simulink model "simulation"  (R2018b)
settings: Solver=FixedStepDiscrete  StartTime=0.0  StopTime=simtime  FixedStep=stepsize  RelTol=1e-3
undefined symbols (not defined in the file): activate_stop, activate_stop_vmax, ay_stop, Bat_param, deltav_ist, DiscIntNeverNeededParam, EG_wunsch, magnitude, mu_road_LF, mu_road_LR, mu_road_RF, mu_road_RR, par_ASR, par_MDT, par_TIR, par_VEH, select_delta_h, select_M_wheel, stepsize, t, temp_betriebsstrategie, temperature_LTrange, track_left, track_right
libraries: Library_ASK x36, simulink x18, dspstat3 x2, Library_Betriebsstrategie x2, vehicle_model x2, pacejka_trans x1
(part 4 of 6)

== system simulation/Vehicle/Antriebsstrang und Radmomentenverteilung/Drehzahlrückführung az VA/Verzögerungsglied ==
  M : Inport
  IC : InitialCondition  Value=0
  PT1_VA : DiscreteTransferFcn  Numerator=par_VEH.dt.other.PT_Num  Denominator=par_VEH.dt.other.PT_Denom
  Zero-Order Hold : ZeroOrderHold  SampleTime=stepsize
  M_d : Outport
  wires:
  IC/1 -> M_d/1
  PT1_VA/1 -> IC/1
  M/1 -> Zero-Order Hold/1
  Zero-Order Hold/1 -> PT1_VA/1

== system simulation/Vehicle/Betriebsstrategie/Momentenverteilung_und_Schaltstrategie1/ASR ==
  Input : Inport
  Limits_In : Inport  Port=2
  mu_road : Inport  Port=3
  Bus Creator : BusCreator  Inputs=10
  Bus Selector : BusSelector  OutputSignals=Fx_RF_ub,Fx_LF_ub,Fx_RR_ub,Fx_LR_ub
  Bus Selector1 : BusSelector  OutputSignals=kappa.kappa_RF,kappa.kappa_LF,kappa.kappa_RR,kappa.kappa_LR
  Bus Selector2 : BusSelector  OutputSignals=x.vx
  Bus Selector3 : BusSelector  OutputSignals=Fz.Fz_RF,Fz.Fz_LF,Fz.Fz_RR,Fz.Fz_LR
  Bus Selector4 : BusSelector  OutputSignals=mu_road_RF,mu_road_LF,mu_road_RR,mu_road_LR
  Bus Selector6 : BusSelector  OutputSignals=Fx_RF_lb,Fx_LF_lb,Fx_RR_lb,Fx_LR_lb,a_f,a_r
  Constant : Constant  Value=0
  Constant1 : Constant  Value=0
  Constant2 : Constant
  Demux : Demux
  Gain : Gain  Gain=500
  Gain1 : Gain  Gain=1/2000
  Gain2 : Gain
  Math Function : Math  Operator=square  SaturateOnIntegerOverflow=on
  Mux : Mux
  Mux1 : Mux
  Mux2 : Mux
  Product : Product
  Saturation1 : Saturate  UpperLimit=1000  LowerLimit=0
  Scope2 : Scope
  Subtract : Sum  Inputs=-+
  Subtract1 : Sum  Inputs=-+
  Switch : Switch  Criteria=u2 > Threshold
  Switch1 : Switch  Criteria=u2 > Threshold
  opt Schlupf : Subsystem
  Limits_Out : Outport
  wires:
  Gain1/1 -> Subtract1/1
  Saturation1/1 -> Gain1/1
  Product/1 -> Demux/1
  Constant1/1 -> Switch1/3
  Switch1/1 -> Saturation1/1
  Bus Selector2/1 -> Switch1/2  "<vx>"
  Math Function/1 -> Switch1/1
  Gain/1 -> Math Function/1
  Switch/1 -> Gain/1
  Constant/1 -> Switch/3
  Bus Selector1/4 -> Mux/4  "<kappa_LR>"
  Bus Selector1/3 -> Mux/3  "<kappa_RR>"
  Bus Selector1/2 -> Mux/2  "<kappa_LF>"
  Bus Selector1/1 -> Mux/1  "<kappa_RF>"
  Limits_In/1 -> Bus Selector/1, Bus Selector6/1
  mu_road/1 -> Bus Selector4/1
  Bus Selector4/1 -> opt Schlupf/1(mu_RF)  "<mu_road_RF>"
  Bus Selector3/1 -> opt Schlupf/5(Fz_RF)  "<Fz_RF>"
  Bus Selector4/2 -> opt Schlupf/2(mu_LF)  "<mu_road_LF>"
  Bus Selector4/3 -> opt Schlupf/3(mu_RR)  "<mu_road_RR>"
  Bus Selector3/2 -> opt Schlupf/6(Fz_LF)  "<Fz_LF>"
  Bus Selector3/4 -> opt Schlupf/8(Fz_LR)  "<Fz_LR>"
  opt Schlupf/1(kappa_soll_RF) -> Mux2/1
  opt Schlupf/2(kappa_soll_LF) -> Mux2/2
  opt Schlupf/3(kappa_soll_RR) -> Mux2/3
  opt Schlupf/4(kappa_soll_LR) -> Mux2/4
  Mux2/1 -> Gain2/1
  Subtract/1 -> Switch/2, Switch/1
  Bus Selector4/4 -> opt Schlupf/4(mu_LR)  "<mu_road_LR>"
  Bus Selector3/3 -> opt Schlupf/7(Fz_RR)  "<Fz_RR>"
  Input/1 -> Bus Selector3/1, Bus Selector2/1, Bus Selector1/1
  Mux/1 -> Subtract/2
  Mux1/1 -> Product/2
  Bus Selector/1 -> Mux1/1  "<Fx_RF_ub>"
  Bus Selector/2 -> Mux1/2  "<Fx_LF_ub>"
  Bus Selector/3 -> Mux1/3  "<Fx_RR_ub>"
  Bus Selector/4 -> Mux1/4  "<Fx_LR_ub>"
  Demux/1 -> Bus Creator/1  "Fx_RF_ub"
  Demux/2 -> Bus Creator/2  "Fx_LF_ub"
  Demux/3 -> Bus Creator/3  "Fx_RR_ub"
  Demux/4 -> Scope2/1, Bus Creator/4  "Fx_LR_ub"
  Bus Selector6/5 -> Bus Creator/9  "<a_f>"
  Bus Selector6/6 -> Bus Creator/10  "<a_r>"
  Bus Creator/1 -> Limits_Out/1
  Subtract1/1 -> Product/1
  Constant2/1 -> Subtract1/2
  Gain2/1 -> Subtract/1
  Bus Selector6/1 -> Bus Creator/5  "<Fx_RF_lb>"
  Bus Selector6/2 -> Bus Creator/6  "<Fx_LF_lb>"
  Bus Selector6/3 -> Bus Creator/7  "<Fx_RR_lb>"
  Bus Selector6/4 -> Bus Creator/8  "<Fx_LR_lb>"

== system simulation/Vehicle/Betriebsstrategie/Momentenverteilung_und_Schaltstrategie1/Feedback Controller ==
  Input : Inport
  Gierrate ref : Inport  Port=2
  Bus Selector2 : BusSelector  OutputSignals=psi.psip
  Feedback control gain : Gain  Gain=par_VEH.tv_control
  Sum : Sum  Inputs=|+-
  M_z_FB : Outport
  wires:
  Bus Selector2/1 -> Sum/2  "<psip>"
  Input/1 -> Bus Selector2/1
  Feedback control gain/1 -> M_z_FB/1
  Sum/1 -> Feedback control gain/1  "error"
  Gierrate ref/1 -> Sum/1

== system simulation/Vehicle/Betriebsstrategie/Momentenverteilung_und_Schaltstrategie1/Feedforward Controller ==
  Input : Inport
  Gierrate ref : Inport  Port=2
  Add : Sum  Inputs=++++
  Add1 : Sum  Inputs=--
  Add2 : Sum
  Add4 : Sum  Inputs=+-
  Add5 : Sum
  Add6 : Sum
  Bus Selector2 : BusSelector  OutputSignals=x.vx,beta.beta,delta_kinematic.delta_RF,delta_kinematic.delta_LF,delta_kinematic.delta_RR,delta_kinematic.delta_LR
  Compare To Zero : simulink/Logic and Bit Operations/Compare To Zero  relop===  OutDataTypeStr=boolean
  Constant1 : Constant  Value=par_VEH.Iz
  Constant10 : Constant  Value=par_VEH.cornering_stiffness_R
  Constant5 : Constant  Value=0
  Constant6 : Constant  Value=0
  Constant7 : Constant  Value=par_VEH.lF
  Constant8 : Constant  Value=par_VEH.lR
  Constant9 : Constant  Value=par_VEH.cornering_stiffness_F
  Discrete Derivative : simulink/Discrete/Discrete Derivative  gainval=1.0  ICPrevScaledInput=0.0  OutMin=[]  OutMax=[]  OutDataType=fixdt(1, 16)  OutScaling=2^-10  DoSatur=off
  Divide{1,6,9..14} (8 alike) : Product  Inputs=**
  Divide7 : Product  Inputs=*/
  Divide8 : Product  Inputs=***
  Gain1 : Gain  Gain=-1
  Gain2 : Gain  Gain=0.5
  Gain3 : Gain  Gain=0.5
  Math Function : Math  Operator=square  SaturateOnIntegerOverflow=on
  Math Function1 : Math  Operator=square  SaturateOnIntegerOverflow=on
  Saturation : Saturate  UpperLimit=1000
  Switch : Switch  Criteria=u2 > Threshold
  M_z_FF : Outport
  wires:
  Input/1 -> Bus Selector2/1
  Gierrate ref/1 -> Divide7/1, Discrete Derivative/1
  Discrete Derivative/1 -> Divide1/2
  Constant1/1 -> Divide1/1
  Divide1/1 -> Divide6/1
  Bus Selector2/1 -> Divide7/2, Compare To Zero/1  "<vx>"
  Constant5/1 -> Divide6/2
  Divide6/1 -> Saturation/1
  Saturation/1 -> Add/1
  Compare To Zero/1 -> Switch/2
  Constant6/1 -> Switch/1
  Divide7/1 -> Switch/3
  Constant9/1 -> Divide12/2, Divide9/2, Divide8/3
  Constant8/1 -> Math Function1/1, Divide10/1
  Constant10/1 -> Divide13/1, Divide10/2
  Bus Selector2/2 -> Divide11/2  "<beta>"
  Divide10/1 -> Add4/2
  Divide9/1 -> Add4/1
  Add4/1 -> Divide11/1
  Constant7/1 -> Math Function/1, Divide9/1, Divide8/2
  Math Function/1 -> Divide12/1
  Math Function1/1 -> Divide13/2
  Divide13/1 -> Add5/2
  Divide12/1 -> Add5/1
  Add5/1 -> Divide14/2
  Switch/1 -> Divide14/1
  Divide14/1 -> Add/4
  Add/1 -> M_z_FF/1
  Divide11/1 -> Add/3
  Gain3/1 -> Add1/1
  Gain2/1 -> Gain1/1
  Add1/1 -> Divide8/1
  Divide8/1 -> Add/2
  Gain1/1 -> Add1/2
  Bus Selector2/5 -> Add2/1  "<delta_RR>"
  Bus Selector2/6 -> Add2/2  "<delta_LR>"
  Add2/1 -> Gain2/1
  Bus Selector2/4 -> Add6/2  "<delta_LF>"
  Add6/1 -> Gain3/1
  Bus Selector2/3 -> Add6/1  "<delta_RF>"

== system simulation/Vehicle/Betriebsstrategie/Momentenverteilung_und_Schaltstrategie1/Gierrate Referenz Berechnung ==
  note: Gewünschte Gierrate nach:
      | psip_desired = vx * delta / (l + vx^2 * K_us )
  input : Inport
  delta_wheel : Inport  Port=2
  2 Räder : Constant  Value=0.5
  Add : Sum
  Bus Selector1 : BusSelector  OutputSignals=delta_RF,delta_LF
  Bus Selector2 : BusSelector  OutputSignals=x.vx
  Constant10 : Constant  Value=par_VEH.l
  Divide : Product  Inputs=*/
  Kus : Constant  Value=EG_wunsch
  Product : Product
  Product1 : Product
  Sum : Sum  Inputs=|++
  delta mittel : Product
  vx^2 : Math  Operator=square  SaturateOnIntegerOverflow=on
  Gierrate ref : Outport
  wires:
  Bus Selector2/1 -> Product/1, vx^2/1  "<vx>"
  input/1 -> Bus Selector2/1
  delta mittel/1 -> Product/2
  2 Räder/1 -> delta mittel/2
  Add/1 -> delta mittel/1
  Bus Selector1/2 -> Add/2  "<delta_LF>"
  Bus Selector1/1 -> Add/1  "<delta_RF>"
  delta_wheel/1 -> Bus Selector1/1
  Divide/1 -> Gierrate ref/1  "Gierrate gewuenscht"
  Product1/1 -> Sum/1
  Sum/1 -> Divide/2
  vx^2/1 -> Product1/1
  Constant10/1 -> Sum/2
  Product/1 -> Divide/1
  Kus/1 -> Product1/2

== system simulation/Vehicle/Betriebsstrategie/Momentenverteilung_und_Schaltstrategie1/Limitierungen gesamt (mit MVS Limits) ==
  Fx_limit : Inport
  M_limit : Inport  Port=2
  M_limit_zentral : Inport  Port=3
  "r_stat_avg " : Inport  Port=4
  Aktuatoren und Delta TV : Subsystem
  Bus Creator : BusCreator  Inputs=10
  Bus Selector : BusSelector  OutputSignals=FxlimRF,FxlimLF,FxlimRR,FxlimLR
  Bus Selector1 : BusSelector  OutputSignals=M_RF_ub,M_RF_lb,M_LF_ub,M_LF_lb,M_RR_ub,M_RR_lb,M_LR_ub,M_LR_lb
  Bus Selector2 : BusSelector  OutputSignals=M_F_lb,M_F_ub,M_R_lb,M_R_ub
  Limits Zusammenführung : MATLAB Function  TreatAsAtomicUnit=on
  Fx_limits : Outport
  wires:
  Aktuatoren und Delta TV/4(A_r) -> Limits Zusammenführung/20(a_r), Bus Creator/10
  Aktuatoren und Delta TV/3(A_f) -> Limits Zusammenführung/19(a_f), Bus Creator/9
  Bus Selector2/4 -> Limits Zusammenführung/16(M_R_ub)  "<M_R_ub>"
  Bus Selector2/3 -> Limits Zusammenführung/15(M_R_lb)  "<M_R_lb>"
  Bus Selector2/2 -> Limits Zusammenführung/14(M_F_ub)  "<M_F_ub>"
  Bus Selector2/1 -> Limits Zusammenführung/13(M_F_lb)  "<M_F_lb>"
  M_limit_zentral/1 -> Bus Selector2/1
  Bus Selector1/8 -> Limits Zusammenführung/12(M_LR_lb)  "<M_LR_lb>"
  Bus Selector1/7 -> Limits Zusammenführung/11(M_LR_ub)  "<M_LR_ub>"
  Bus Selector1/6 -> Limits Zusammenführung/10(M_RR_lb)  "<M_RR_lb>"
  Bus Selector1/5 -> Limits Zusammenführung/9(M_RR_ub)  "<M_RR_ub>"
  Bus Selector1/4 -> Limits Zusammenführung/8(M_LF_lb)  "<M_LF_lb>"
  Bus Selector1/3 -> Limits Zusammenführung/7(M_LF_ub)  "<M_LF_ub>"
  Bus Selector1/2 -> Limits Zusammenführung/6(M_RF_lb)  "<M_RF_lb>"
  Bus Selector1/1 -> Limits Zusammenführung/5(M_RF_ub)  "<M_RF_ub>"
  Bus Selector/4 -> Limits Zusammenführung/4(FxlimLR)  "<FxlimLR>"
  Bus Selector/3 -> Limits Zusammenführung/3(FxlimRR)  "<FxlimRR>"
  Bus Selector/2 -> Limits Zusammenführung/2(FxlimLF)  "<FxlimLF>"
  Bus Selector/1 -> Limits Zusammenführung/1(FxlimRF)  "<FxlimRF>"
  Bus Creator/1 -> Fx_limits/1
  M_limit/1 -> Bus Selector1/1
  Fx_limit/1 -> Bus Selector/1
  "r_stat_avg "/1 -> Limits Zusammenführung/21(r)
  Aktuatoren und Delta TV/1(Delta_T_f) -> Limits Zusammenführung/17(DELTA_T_f)
  Aktuatoren und Delta TV/2(Delta_T_r) -> Limits Zusammenführung/18(DELTA_T_r)
  Limits Zusammenführung/1(Fx_LF_ub) -> Bus Creator/1  "Fx_LF_ub"
  Limits Zusammenführung/2(Fx_LF_lb) -> Bus Creator/2  "Fx_LF_lb"
  Limits Zusammenführung/3(Fx_RF_ub) -> Bus Creator/3  "Fx_RF_ub"
  Limits Zusammenführung/4(Fx_RF_lb) -> Bus Creator/4  "Fx_RF_lb"
  Limits Zusammenführung/5(Fx_LR_ub) -> Bus Creator/5  "Fx_LR_ub"
  Limits Zusammenführung/6(Fx_LR_lb) -> Bus Creator/6  "Fx_LR_lb"
  Limits Zusammenführung/7(Fx_RR_ub) -> Bus Creator/7  "Fx_RR_ub"
  Limits Zusammenführung/8(Fx_RR_lb) -> Bus Creator/8  "Fx_RR_lb"

== system simulation/Vehicle/Betriebsstrategie/Momentenverteilung_und_Schaltstrategie1/Momente für die Reibbremse ==
  M_antr : Inport
  M_wheel : Inport  Port=2
  v_x : Inport  Port=3
  Add : Sum  Inputs=-+
  Add1 : Sum  Inputs=++++
  Bias : Bias  Bias=-1
  Bus Creator1 : BusCreator  Inputs=4
  Bus Selector : BusSelector  OutputSignals=M_antr_LF,M_antr_LR,M_antr_RF,M_antr_RR
  Constant1 : Constant  Value=par_VEH.bkv
  Product4 : Product  Inputs=3
  Product5 : Product  Inputs=3
  Saturation2 : Saturate  UpperLimit=0  LowerLimit=-5000
  Sign : Signum
  Signal Conversion : SignalConversion  OverrideOpt=off
  Signal Conversion1 : SignalConversion  OverrideOpt=off
  Unary Minus : UnaryMinus
  Unit Delay2 : UnitDelay  InitialCondition=2  SampleTime=-1
  M_brems : Outport
  wires:
  Signal Conversion1/1 -> Bus Creator1/4  "M_brems_RR"
  Product5/1 -> Bus Creator1/3, Signal Conversion1/1  "M_brems_RF"
  Signal Conversion/1 -> Bus Creator1/2  "M_brems_LR"
  Product4/1 -> Signal Conversion/1, Bus Creator1/1  "M_brems_LF"
  Bus Creator1/1 -> M_brems/1
  Bus Selector/1 -> Add1/1  "<M_antr_LF>"
  Bus Selector/2 -> Add1/2  "<M_antr_LR>"
  Bus Selector/3 -> Add1/3  "<M_antr_RF>"
  Bus Selector/4 -> Add1/4  "<M_antr_RR>"
  M_antr/1 -> Bus Selector/1
  v_x/1 -> Unit Delay2/1
  Constant1/1 -> Bias/1, Product4/1
  Unit Delay2/1 -> Sign/1
  Sign/1 -> Product5/3, Product4/3
  Unary Minus/1 -> Product5/2
  Bias/1 -> Unary Minus/1
  Saturation2/1 -> Product4/2, Product5/1
  Add/1 -> Saturation2/1
  M_wheel/1 -> Add/2
  Add1/1 -> Add/1

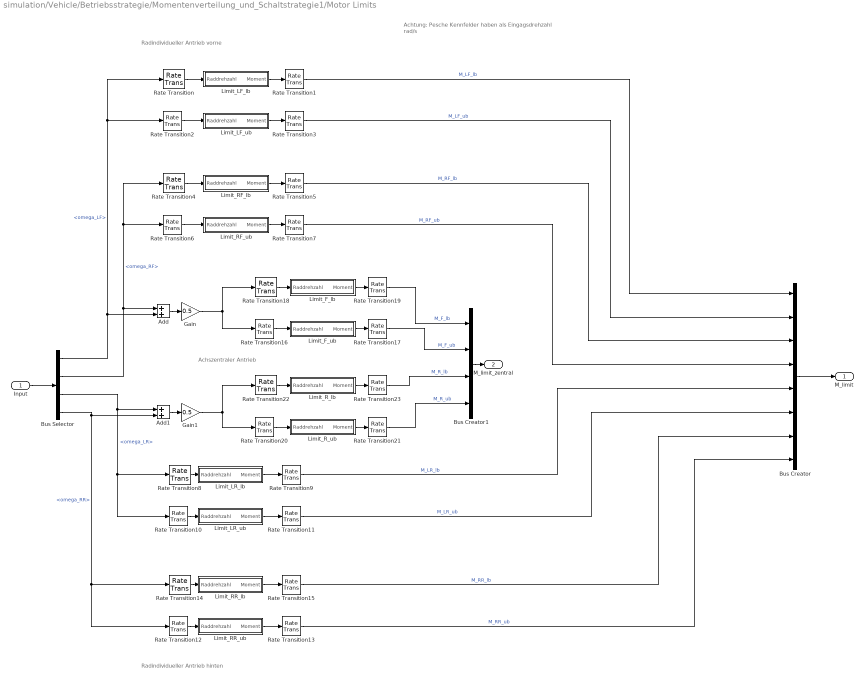
== system simulation/Vehicle/Betriebsstrategie/Momentenverteilung_und_Schaltstrategie1/Motor Limits ==
  note: Achtung:
      | Pesche Kennfelder haben als Eingagsdrehzahl rad/s
  note: Radindividueller Antrieb vorne
  note: Radindividueller Antrieb hinten
  note: Achszentraler Antrieb
  Input : Inport
  Add : Sum
  Add1 : Sum
  Bus Creator : BusCreator  Inputs=8
  Bus Creator1 : BusCreator  Inputs=4
  Bus Selector : BusSelector  OutputSignals=omega.omega_LF,omega.omega_RF,omega.omega_LR,omega.omega_RR
  Gain : Gain  Gain=0.5
  Gain1 : Gain  Gain=0.5
  Limit_F_lb : Subsystem
  Limit_F_ub : Subsystem
  Limit_LF_lb : Subsystem
  Limit_LF_ub : Subsystem
  Limit_LR_lb : Subsystem
  Limit_LR_ub : Subsystem
  Limit_RF_lb : Subsystem
  Limit_RF_ub : Subsystem
  Limit_RR_lb : Subsystem
  Limit_RR_ub : Subsystem
  Limit_R_lb : Subsystem
  Limit_R_ub : Subsystem
  Rate Transition{,2,4,6,8,10,12,14,16,18,20,22} (12 alike) : RateTransition  OutPortSampleTime=stepsize*10
  Rate Transition{1,3,5,7,9,11,13,15,17,19,21,23} (12 alike) : RateTransition  OutPortSampleTimeOpt=Inherit  OutPortSampleTime=0.001
  M_limit : Outport
  M_limit_zentral : Outport  Port=2
  wires:
  Rate Transition/1 -> Limit_LF_lb/1(Raddrehzahl)
  Rate Transition21/1 -> Bus Creator1/4  "M_R_ub"
  Rate Transition23/1 -> Bus Creator1/3  "M_R_lb"
  Rate Transition19/1 -> Bus Creator1/1  "M_F_lb"
  Gain1/1 -> Rate Transition22/1, Rate Transition20/1
  Add1/1 -> Gain1/1
  Gain/1 -> Rate Transition18/1, Rate Transition16/1
  Add/1 -> Gain/1
  Rate Transition22/1 -> Limit_R_lb/1(Raddrehzahl)
  Rate Transition20/1 -> Limit_R_ub/1(Raddrehzahl)
  Rate Transition18/1 -> Limit_F_lb/1(Raddrehzahl)
  Rate Transition16/1 -> Limit_F_ub/1(Raddrehzahl)
  Bus Selector/4 -> Rate Transition14/1, Rate Transition12/1, Add1/2  "<omega_RR>"
  Bus Selector/3 -> Rate Transition10/1, Rate Transition8/1, Add1/1  "<omega_LR>"
  Rate Transition14/1 -> Limit_RR_lb/1(Raddrehzahl)
  Rate Transition12/1 -> Limit_RR_ub/1(Raddrehzahl)
  Rate Transition8/1 -> Limit_LR_lb/1(Raddrehzahl)
  Rate Transition10/1 -> Limit_LR_ub/1(Raddrehzahl)
  Bus Selector/2 -> Add/1, Rate Transition4/1, Rate Transition6/1  "<omega_RF>"
  Rate Transition4/1 -> Limit_RF_lb/1(Raddrehzahl)
  Rate Transition6/1 -> Limit_RF_ub/1(Raddrehzahl)
  Bus Selector/1 -> Rate Transition/1, Rate Transition2/1, Add/2  "<omega_LF>"
  Rate Transition2/1 -> Limit_LF_ub/1(Raddrehzahl)
  Input/1 -> Bus Selector/1
  Rate Transition3/1 -> Bus Creator/2  "M_LF_ub"
  Rate Transition5/1 -> Bus Creator/3  "M_RF_lb"
  Rate Transition7/1 -> Bus Creator/4  "M_RF_ub"
  Rate Transition1/1 -> Bus Creator/1  "M_LF_lb"
  Rate Transition9/1 -> Bus Creator/5  "M_LR_lb"
  Rate Transition11/1 -> Bus Creator/6  "M_LR_ub"
  Rate Transition15/1 -> Bus Creator/7  "M_RR_lb"
  Rate Transition13/1 -> Bus Creator/8  "M_RR_ub"
  Bus Creator/1 -> M_limit/1
  Bus Creator1/1 -> M_limit_zentral/1
  Rate Transition17/1 -> Bus Creator1/2  "M_F_ub"
  Limit_RR_ub/1(Moment) -> Rate Transition13/1
  Limit_RR_lb/1(Moment) -> Rate Transition15/1
  Limit_LR_ub/1(Moment) -> Rate Transition11/1
  Limit_LR_lb/1(Moment) -> Rate Transition9/1
  Limit_R_lb/1(Moment) -> Rate Transition23/1
  Limit_R_ub/1(Moment) -> Rate Transition21/1
  Limit_LF_lb/1(Moment) -> Rate Transition1/1
  Limit_LF_ub/1(Moment) -> Rate Transition3/1
  Limit_RF_lb/1(Moment) -> Rate Transition5/1
  Limit_RF_ub/1(Moment) -> Rate Transition7/1
  Limit_F_lb/1(Moment) -> Rate Transition19/1
  Limit_F_ub/1(Moment) -> Rate Transition17/1

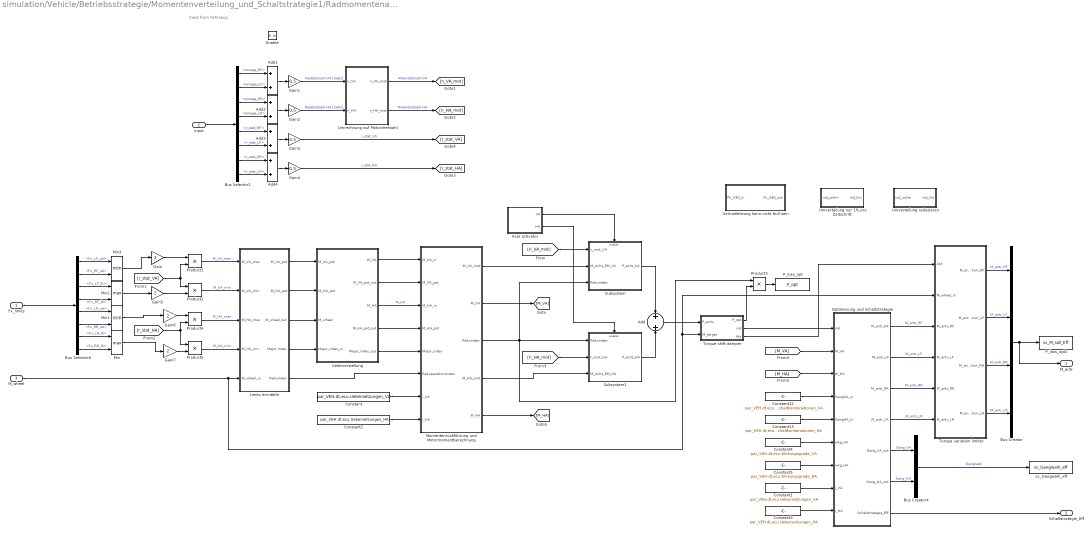
== system simulation/Vehicle/Betriebsstrategie/Momentenverteilung_und_Schaltstrategie1/Radmomentenaufteilung (Effizienz) ==
  note: Input from Fahrzeug
  Fx_limits : Inport
  Input : Inport  Port=2
  M_wheel : Inport  Port=3
  Enable : EnablePort
  Add{,1..4} (5 alike) : Sum
  Axle activator : Subsystem
  Bus Creator : BusCreator  Inputs=4
  Bus Creator4 : BusCreator  Inputs=2
  Bus Selector2 : BusSelector  OutputSignals=omega.omega_RF,omega.omega_LF,omega.omega_RR,omega.omega_LR,r_stat.r_stat_RF,r_stat.r_stat_LF,r_stat.r_stat_RR,r_stat.r_stat_LR
  Bus Selector6 : BusSelector  OutputSignals=Fx_LF_ub,Fx_RF_ub,Fx_LF_lb,Fx_RF_lb,Fx_LR_ub,Fx_RR_ub,Fx_LR_lb,Fx_RR_lb
  Constant : Constant  Value=par_VEH.dt.ecu.Uebersetzungen_VA
  Constant1 : Constant  Value=par_VEH.dt.ecu.Uebersetzungen_VA
  Constant12 : Constant  Value=par_VEH.dt.ecu.Schaltkombinationen_VA
  Constant13 : Constant  Value=par_VEH.dt.ecu.Schaltkombinationen_HA
  Constant2 : Constant  Value=par_VEH.dt.ecu.Uebersetzungen_HA
  Constant3 : Constant  Value=par_VEH.dt.ecu.Uebersetzungen_HA
  Constant4 : Constant  Value=par_VEH.dt.ecu.Wirkungsgrade_VA
  Constant5 : Constant  Value=par_VEH.dt.ecu.Wirkungsgrade_HA
  Gain{,5..7} (4 alike) : Gain  Gain=2
  Gain{1..4} (4 alike) : Gain  Gain=0.5
  Limits ermitteln : Subsystem
  Min : MinMax  Function=max  Inputs=2
  Min1 : MinMax  Inputs=2
  Min2 : MinMax  Function=max  Inputs=2
  Min3 : MinMax  Inputs=2
  Momentenrückführung und Motormomentberechnung : Subsystem
  Optimierung und Schaltstrategie : Subsystem
  P_loss_opt : ToWorkspace  VariableName=P_opt  SampleTime=-1
      settings: Decimation=savedec
  P_loss_opt1 : ToWorkspace  VariableName=sv_M_soll_Eff  SampleTime=-1
      settings: Decimation=savedec
  Product{1..5} (5 alike) : Product
  Subsystem : Subsystem
  Subsystem1 : Subsystem
  Torque shift damper : Subsystem
  Torque variation limiter : Subsystem
  Umrechnung auf Motordrehzahl : Subsystem
  Umverteilung nur 1% pro Zeitschritt : Subsystem
  Umverteilung reduzieren : Subsystem
  Vektorerstellung : Subsystem
  Verlustleistung kann nicht Null sein : Subsystem
  sv_Gangwahl_eff : ToWorkspace  VariableName=sv_Gangwahl_eff  SaveFormat=Timeseries  SampleTime=-1
      settings: Decimation=savedec
  M_antr : Outport
  Schaltstrategie_Eff : Outport  Port=2
  wires:
  Fx_limits/1 -> Bus Selector6/1
  Bus Selector6/7 -> Min/1  "<Fx_LR_lb>"
  Bus Selector6/8 -> Min/2  "<Fx_RR_lb>"
  Bus Selector6/5 -> Min1/1  "<Fx_LR_ub>"
  Bus Selector6/6 -> Min1/2  "<Fx_RR_ub>"
  Bus Selector6/4 -> Min2/2  "<Fx_RF_lb>"
  Bus Selector6/2 -> Min3/2  "<Fx_RF_ub>"
  Bus Selector6/3 -> Min2/1  "<Fx_LF_lb>"
  Bus Selector6/1 -> Min3/1  "<Fx_LF_ub>"
  Input/1 -> Bus Selector2/1
  Add1/1 -> Gain1/1
  Bus Selector2/1 -> Add1/1  "<omega_RF>"
  Bus Selector2/2 -> Add1/2  "<omega_LF>"
  Add2/1 -> Gain2/1
  Bus Selector2/3 -> Add2/1  "<omega_RR>"
  Bus Selector2/4 -> Add2/2  "<omega_LR>"
  Gain1/1 -> Umrechnung auf Motordrehzahl/1(n_VA)  "Raddrehzahl VA [rad/s]"
  Gain2/1 -> Umrechnung auf Motordrehzahl/2(n_HA)  "Raddrehzahl HA [rad/s]"
  Add3/1 -> Gain3/1
  Add4/1 -> Gain4/1
  Bus Selector2/8 -> Add4/2  "<r_stat_LR>"
  Bus Selector2/6 -> Add3/2  "<r_stat_LF>"
  Bus Selector2/5 -> Add3/1  "<r_stat_RF>"
  Bus Selector2/7 -> Add4/1  "<r_stat_RR>"
  Gain4/1 -> [r_stat_HA]  "r_stat_HA"
  Gain3/1 -> [r_stat_VA]  "r_stat_VA"
  Limits ermitteln/3(M_wheel_out) -> Vektorerstellung/3(M_wheel)
  Vektorerstellung/3(M_HA) -> Momentenrückführung und Motormomentberechnung/3(M_HA_in)  "M_HA"
  Umrechnung auf Motordrehzahl/1(n_VA_mot) -> [n_VA_mot]  "Motordrehzahl VA"
  Umrechnung auf Motordrehzahl/2(n_HA_mot) -> [n_HA_mot]  "Motordrehzahl HA"
  Constant/1 -> Momentenrückführung und Motormomentberechnung/7(i_VA)
  Constant2/1 -> Momentenrückführung und Motormomentberechnung/8(i_HA)
  Limits ermitteln/5(Rekuindex) -> Momentenrückführung und Motormomentberechnung/6(Rekuperationsindex)
  Vektorerstellung/1(M_VA) -> Momentenrückführung und Motormomentberechnung/1(M_VA_in)
  Limits ermitteln/1(M_VA_pot) -> Vektorerstellung/1(M_VA_pot)
  Limits ermitteln/2(M_HA_pot) -> Vektorerstellung/2(M_HA_pot)
  Vektorerstellung/2(M_VA_pot_out) -> Momentenrückführung und Motormomentberechnung/2(M_VA_pot)
  Vektorerstellung/4(M_HA_pot_out) -> Momentenrückführung und Motormomentberechnung/4(M_HA_pot)
  Bus Creator4/1 -> sv_Gangwahl_eff/1  "Gangwahl"
  Constant12/1 -> Optimierung und Schaltstrategie/4(GangVA_in)
  Bus Creator/1 -> M_antr/1, P_loss_opt1/1
  Torque variation limiter/1(M_antr_korr_RF) -> Bus Creator/1  "M_antr_RF"
  Torque variation limiter/2(M_antr_korr_LF) -> Bus Creator/2  "M_antr_LF"
  Torque variation limiter/3(M_antr_korr_RR) -> Bus Creator/3  "M_antr_RR"
  Torque variation limiter/4(M_antr_korr_LR) -> Bus Creator/4  "M_antr_LR"
  Optimierung und Schaltstrategie/5(Gang_VA_out) -> Bus Creator4/1  "Gang_VA"
  Constant13/1 -> Optimierung und Schaltstrategie/5(GangHA_in)
  Optimierung und Schaltstrategie/6(Gang_HA_out) -> Bus Creator4/2  "Gang_HA"
  Optimierung und Schaltstrategie/7(Schaltstrategie_Eff) -> Schaltstrategie_Eff/1
  Constant5/1 -> Optimierung und Schaltstrategie/7(wkg_HA)
  Constant4/1 -> Optimierung und Schaltstrategie/6(wkg_VA)
  Constant3/1 -> Optimierung und Schaltstrategie/9(i_HA)
  Constant1/1 -> Optimierung und Schaltstrategie/8(i_VA)
  Momentenrückführung und Motormomentberechnung/2(M_VA) -> [M_VA]
  Momentenrückführung und Motormomentberechnung/3(Rekuindex) -> Subsystem/3(Rekuindex), Product3/1, Subsystem1/1(Rekuindex)
  Add/1 -> Torque shift damper/1(P_achs)
  Momentenrückführung und Motormomentberechnung/5(M_HA) -> [M_HA]
  Product3/1 -> P_loss_opt/1
  [M_VA] -> Optimierung und Schaltstrategie/2(M_VA)
  [M_HA] -> Optimierung und Schaltstrategie/3(M_HA)
  Product2/1 -> Limits ermitteln/2(M_VA_min)  "M_VA_min"
  [r_stat_VA] -> Product1/2, Product2/1
  Min/1 -> Gain7/1
  Min3/1 -> Gain/1
  Gain5/1 -> Product2/2
  Min2/1 -> Gain5/1
  Gain6/1 -> Product4/1
  Min1/1 -> Gain6/1
  [r_stat_HA] -> Product4/2, Product5/1
  Gain7/1 -> Product5/2
  Gain/1 -> Product1/1
  Product4/1 -> Limits ermitteln/3(M_HA_max)  "M_HA_max"
  Product1/1 -> Limits ermitteln/1(M_VA_max)  "M_VA_max"
  Product5/1 -> Limits ermitteln/4(M_HA_min)  "M_HA_min"
  Torque shift damper/3(Akt) -> Torque variation limiter/1(Akt)
  M_wheel/1 -> Torque shift damper/2(M_target), Torque variation limiter/2(M_wheel_in), Limits ermitteln/5(M_wheel_in)
  Optimierung und Schaltstrategie/1(M_antr_RF) -> Torque variation limiter/3(M_antr_RF)  "M_antr_RF"
  Optimierung und Schaltstrategie/2(M_antr_LF) -> Torque variation limiter/4(M_antr_LF)  "M_antr_LF"
  Optimierung und Schaltstrategie/3(M_antr_RR) -> Torque variation limiter/5(M_antr_RR)  "M_antr_RR"
  Optimierung und Schaltstrategie/4(M_antr_LR) -> Torque variation limiter/6(M_antr_LR)  "M_antr_LR"
  Limits ermitteln/4(Major index) -> Vektorerstellung/4(Major_index_in)
  Vektorerstellung/5(Major_index_out) -> Momentenrückführung und Motormomentberechnung/5(Major_index)
  [n_VA_mot] -> Subsystem/1(n_mot_VA)
  Subsystem/1(P_achs_VA) -> Add/1
  [n_HA_mot] -> Subsystem1/2(n_mot_HA)
  Subsystem1/1(P_achs_HA) -> Add/2
  Axle activator/1(VA) -> Subsystem/Enable
  Axle activator/2(HA) -> Subsystem1/Enable
  Momentenrückführung und Motormomentberechnung/1(M_VA_mot) -> Subsystem/2(M_Achs_EM_VA)
  Momentenrückführung und Motormomentberechnung/4(M_HA_mot) -> Subsystem1/3(M_Achs_EM_HA)
  Torque shift damper/1(P_opt) -> Product3/2
  Torque shift damper/2(ind) -> Optimierung und Schaltstrategie/1(ind)

== system simulation/Vehicle/Betriebsstrategie/Momentenverteilung_und_Schaltstrategie1/Radmomentenaufteilung (Standardfahrmanöver) ==
  Fx_limits : Inport
  Input : Inport  Port=2
  M_z_desired : Inport  Port=3
  M_wheel : Inport  Port=4
  Delta_wheel : Inport  Port=5
  Enable : EnablePort
  Abs : Abs
  Add : Sum
  Bus Creator : BusCreator  Inputs=4
  Bus Selector1 : BusSelector  OutputSignals=delta_RF,delta_LF
  Bus Selector4 : BusSelector  OutputSignals=Fx_LF_ub,Fx_LF_lb,Fx_RF_ub,Fx_RF_lb,Fx_LR_ub,Fx_LR_lb,Fx_RR_ub,Fx_RR_lb,a_f,a_r
  Bus Selector5 : BusSelector  OutputSignals=a_f,a_r
  Constant1 : Constant  Value=par_VEH.sR
  Constant10 : Constant  Value=par_VEH.sF
  Constant2 : Constant  Value=par_VEH.lR
  Constant24 : Constant  Value=par_VEH.lF
  Gain4 : Gain  Gain=0.5
  Limit : simulink/Discontinuities/Saturation Dynamic  OutMin=[]  OutMax=[]  OutDataTypeStr=Inherit: Same as second input  OutDataType=fixdt(1, 16)  OutScaling=2^-10  DoSatur=off
  Limits : Subsystem
  Limits berücksichtigen : MATLAB Function  TreatAsAtomicUnit=on
  Lo : Gain  Gain=-1
  Memory{,1..3} (4 alike) : Memory
  MomentForce : Subsystem
  MomentForce1 : Subsystem
  Optimierung mit Lagrange Multiplikator Methode : MATLAB Function  TreatAsAtomicUnit=on
  Schaltstrategie : Subsystem
  M_antr : Outport
  Schaltstrategie_Dyn : Outport  Port=2
  wires:
  Input/1 -> MomentForce/1(Input), MomentForce1/5(Input), Schaltstrategie/2(From Fahrzeugmodell)
  Memory3/1 -> Optimierung mit Lagrange Multiplikator Methode/14(X_FL1)
  Memory2/1 -> Optimierung mit Lagrange Multiplikator Methode/15(X_FR1)
  Memory/1 -> Optimierung mit Lagrange Multiplikator Methode/17(X_RR1)
  Optimierung mit Lagrange Multiplikator Methode/4(X_RR) -> Limits berücksichtigen/14(X_RR), Memory/1
  Optimierung mit Lagrange Multiplikator Methode/2(X_FR) -> Limits berücksichtigen/12(X_FR), Memory2/1
  Gain4/1 -> Optimierung mit Lagrange Multiplikator Methode/13(delta)
  Add/1 -> Gain4/1
  Bus Selector1/2 -> Add/2  "<delta_LF>"
  Bus Selector1/1 -> Add/1  "<delta_RF>"
  Delta_wheel/1 -> Bus Selector1/1
  Constant2/1 -> Optimierung mit Lagrange Multiplikator Methode/12(lr)
  Constant24/1 -> Optimierung mit Lagrange Multiplikator Methode/11(lf)
  Constant1/1 -> Optimierung mit Lagrange Multiplikator Methode/10(tR)
  Constant10/1 -> Optimierung mit Lagrange Multiplikator Methode/9(tF)
  MomentForce1/4(M_antr_LR) -> Bus Creator/4  "M_antr_LR"
  MomentForce1/3(M_antr_RR) -> Bus Creator/3  "M_antr_RR"
  MomentForce1/2(M_antr_LF) -> Bus Creator/2  "M_antr_LF"
  MomentForce1/1(M_antr_RF) -> Bus Creator/1  "M_antr_RF"
  Bus Creator/1 -> M_antr/1, Schaltstrategie/1(Drehmomente am Rad)
  Memory1/1 -> Optimierung mit Lagrange Multiplikator Methode/16(X_RL1)
  Bus Selector4/1 -> Limits berücksichtigen/1(Fx_LF_ub)  "<Fx_LF_ub>"
  Bus Selector4/2 -> Limits berücksichtigen/2(Fx_LF_lb)  "<Fx_LF_lb>"
  Bus Selector4/3 -> Limits berücksichtigen/3(Fx_RF_ub)  "<Fx_RF_ub>"
  Bus Selector4/4 -> Limits berücksichtigen/4(Fx_RF_lb)  "<Fx_RF_lb>"
  Bus Selector4/5 -> Limits berücksichtigen/5(Fx_LR_ub)  "<Fx_LR_ub>"
  Bus Selector4/6 -> Limits berücksichtigen/6(Fx_LR_lb)  "<Fx_LR_lb>"
  Bus Selector4/7 -> Limits berücksichtigen/7(Fx_RR_ub)  "<Fx_RR_ub>"
  Bus Selector4/8 -> Limits berücksichtigen/8(Fx_RR_lb)  "<Fx_RR_lb>"
  Bus Selector4/9 -> Limits berücksichtigen/9(a_f)  "<a_f>"
  Bus Selector4/10 -> Limits berücksichtigen/10(a_r)  "<a_r>"
  Optimierung mit Lagrange Multiplikator Methode/3(X_RL) -> Limits berücksichtigen/13(X_RL), Memory1/1
  Fx_limits/1 -> Limits/1(Limits), Bus Selector5/1, Bus Selector4/1
  Bus Selector5/1 -> Optimierung mit Lagrange Multiplikator Methode/1(a_f)  "<a_f>"
  Bus Selector5/2 -> Optimierung mit Lagrange Multiplikator Methode/2(a_r)  "<a_r>"
  Limits berücksichtigen/1(Fx_RF) -> MomentForce1/1(Fx_RF)
  Limits berücksichtigen/2(Fx_LF) -> MomentForce1/2(Fx_LF)
  Limits berücksichtigen/3(Fx_RR) -> MomentForce1/3(Fx_RR)
  Limits berücksichtigen/4(Fx_LR) -> MomentForce1/4(Fx_LR)
  Schaltstrategie/1(SchaltstrategieOut) -> Schaltstrategie_Dyn/1
  M_wheel/1 -> MomentForce/2(MWheel), Limits/2(M_wheel)
  MomentForce/1(XWheel) -> Limit/2
  Limits/2(Limit_FL) -> Optimierung mit Lagrange Multiplikator Methode/4(Z_FL)
  Limits/3(Limit_FR) -> Optimierung mit Lagrange Multiplikator Methode/5(Z_FR)
  Limits/4(Limit_RL) -> Optimierung mit Lagrange Multiplikator Methode/6(Z_RL)
  Limits/5(Limit_RR) -> Optimierung mit Lagrange Multiplikator Methode/7(Z_RR)
  Limit/1 -> Optimierung mit Lagrange Multiplikator Methode/3(X_req)
  Limits/1(X_Max) -> Abs/1
  Lo/1 -> Limit/3
  Abs/1 -> Lo/1, Limit/1
  M_z_desired/1 -> Optimierung mit Lagrange Multiplikator Methode/8(Mz)
  Optimierung mit Lagrange Multiplikator Methode/1(X_FL) -> Limits berücksichtigen/11(X_FL), Memory3/1

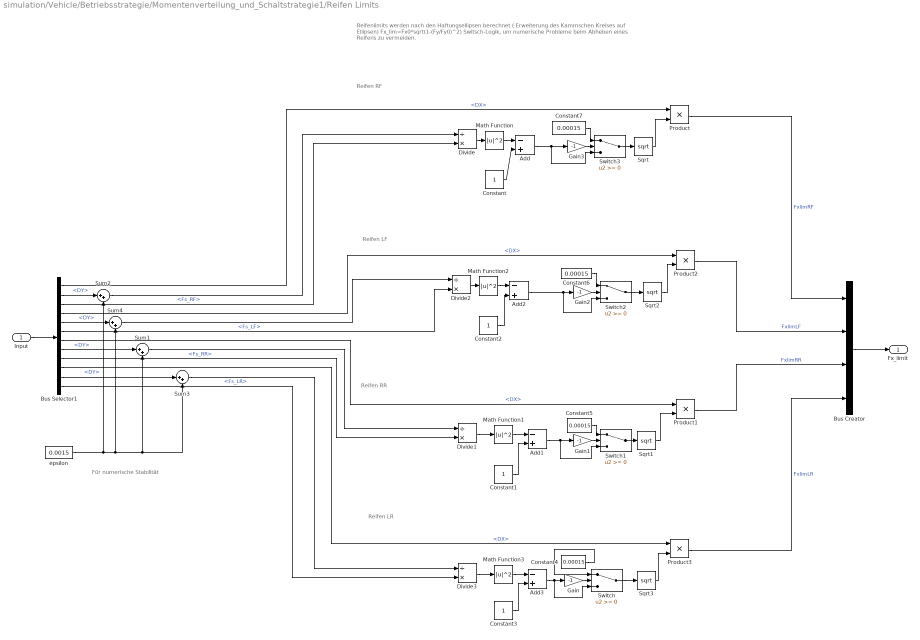
== system simulation/Vehicle/Betriebsstrategie/Momentenverteilung_und_Schaltstrategie1/Reifen Limits ==
  note: Reifen RF
  note: Reifen LF
  note: Reifen RR
  note: Reifen LR
  note: Für numerische Stabilität
  note: Reifenlimits werden nach den Haftungsellipsen berechnet ( Erweiterung des Kammschen Kreises auf Ellipsen)
      | Fx_lim=Fx0*sqrt(1-(Fy/Fy0)^2)
      |
      | Switsch-Logik, um numerische Probleme beim Abheben eines Reifens zu vermeiden.
  Input : Inport
  Add{,1..3} (4 alike) : Sum  Inputs=-+
  Bus Creator : BusCreator  Inputs=4
  Bus Selector1 : BusSelector  OutputSignals=F0.RF.DX,F0.RF.DY,Fs.Fs_RF,F0.LF.DX,F0.LF.DY,Fs.Fs_LF,F0.RR.DX,F0.RR.DY,Fs.Fs_RR,F0.LR.DX,F0.LR.DY,Fs.Fs_LR
  Constant{,1..3} (4 alike) : Constant
  Constant{4..7} (4 alike) : Constant  Value=0.00015
  Divide{,1..3} (4 alike) : Product  Inputs=/*
  Gain{,1..3} (4 alike) : Gain  Gain=-1
  Math Function{,1..3} (4 alike) : Math  Operator=magnitude^2  SaturateOnIntegerOverflow=on
  Product{,1..3} (4 alike) : Product
  Sqrt{,1..3} (4 alike) : Sqrt  SaturateOnIntegerOverflow=on
  Sum{1..4} (4 alike) : Sum  Inputs=|++
  Switch{,1..3} (4 alike) : Switch
  epsilon : Constant  Value=0.0015
  Fx_limit : Outport
  wires:
  Bus Selector1/10 -> Product3/1  "<DX>"
  Bus Selector1/5 -> Sum4/1  "<DY>"
  Bus Selector1/8 -> Sum1/1  "<DY>"
  Bus Selector1/11 -> Sum3/1  "<DY>"
  Bus Selector1/2 -> Sum2/1  "<DY>"
  epsilon/1 -> Sum3/2, Sum1/2, Sum4/2, Sum2/2
  Bus Selector1/1 -> Product/1  "<DX>"
  Sum2/1 -> Divide/1
  Math Function/1 -> Add/1
  Constant/1 -> Add/2
  Sqrt/1 -> Product/2
  Bus Selector1/7 -> Product1/1  "<DX>"
  Sum1/1 -> Divide1/1
  Divide1/1 -> Math Function1/1
  Math Function1/1 -> Add1/1
  Constant1/1 -> Add1/2
  Sqrt1/1 -> Product1/2
  Bus Selector1/4 -> Product2/1  "<DX>"
  Sum4/1 -> Divide2/1
  Divide2/1 -> Math Function2/1
  Math Function2/1 -> Add2/1
  Constant2/1 -> Add2/2
  Sqrt2/1 -> Product2/2
  Sum3/1 -> Divide3/1
  Divide3/1 -> Math Function3/1
  Math Function3/1 -> Add3/1
  Constant3/1 -> Add3/2
  Sqrt3/1 -> Product3/2
  Divide/1 -> Math Function/1
  Input/1 -> Bus Selector1/1
  Bus Selector1/3 -> Divide/2  "<Fs_RF>"
  Bus Selector1/6 -> Divide2/2  "<Fs_LF>"
  Bus Selector1/9 -> Divide1/2  "<Fs_RR>"
  Bus Selector1/12 -> Divide3/2  "<Fs_LR>"
  Product/1 -> Bus Creator/1  "FxlimRF"
  Product2/1 -> Bus Creator/2  "FxlimLF"
  Product1/1 -> Bus Creator/3  "FxlimRR"
  Product3/1 -> Bus Creator/4  "FxlimLR"
  Bus Creator/1 -> Fx_limit/1
  Add3/1 -> Switch/3, Gain/1
  Gain/1 -> Switch/2
  Constant4/1 -> Switch/1
  Switch/1 -> Sqrt3/1
  Add1/1 -> Gain1/1, Switch1/3
  Gain1/1 -> Switch1/2
  Constant5/1 -> Switch1/1
  Switch1/1 -> Sqrt1/1
  Add2/1 -> Switch2/3, Gain2/1
  Gain2/1 -> Switch2/2
  Constant6/1 -> Switch2/1
  Switch2/1 -> Sqrt2/1
  Add/1 -> Gain3/1, Switch3/3
  Gain3/1 -> Switch3/2
  Constant7/1 -> Switch3/1
  Switch3/1 -> Sqrt/1

== system simulation/Vehicle/Betriebsstrategie/Momentenverteilung_und_Schaltstrategie1/Reifenradius  ==
  Input : Inport
  Add : Sum  Inputs=++++
  Bus Selector1 : BusSelector  OutputSignals=r_stat.r_stat_RF,r_stat.r_stat_LF,r_stat.r_stat_RR,r_stat.r_stat_LR
  Gain : Gain  Gain=1/4
  IC : InitialCondition  Value=par_VEH.r_stat0
  r_stat_avg : Outport
  wires:
  Bus Selector1/1 -> Add/1  "<r_stat_RF>"
  Bus Selector1/4 -> Add/4  "<r_stat_LR>"
  Input/1 -> Bus Selector1/1
  Bus Selector1/2 -> Add/2  "<r_stat_LF>"
  Add/1 -> Gain/1
  Gain/1 -> IC/1
  Bus Selector1/3 -> Add/3  "<r_stat_RR>"
  IC/1 -> r_stat_avg/1

== system simulation/Vehicle/Betriebsstrategie/Momentenverteilung_und_Schaltstrategie1/adaptive Limiter ==
  Input : Inport
  M_z_FB : Inport  Port=2
  M_z_FF : Inport  Port=3
  1-D Lookup Table : Lookup_n-D  NumberOfTableDimensions=1  BreakpointsForDimension1=[-10,-9,-8.5,-8,-7.5,7.5,8,8.5,9,10]  Table=[0,0,0.5,0.9,1,1,0.9,0.5,0,0]  ExtrapMethod=Clip  UseLastTableValue=on  InternalRulePriority=Speed  RndMeth=Simplest  InputSameDT=on
  1-D Lookup Table1 : Lookup_n-D  NumberOfTableDimensions=1  BreakpointsForDimension1=[-10,-9,-8,-7.5,7.5,8,9,10]  Table=[0.3,0.12,0.03,0,0,0.03,0.12,0.3]  ExtrapMethod=Clip  UseLastTableValue=on  InternalRulePriority=Speed  RndMeth=Simplest  InputSameDT=on
  1-D Lookup Table2 : Lookup_n-D  NumberOfTableDimensions=1  BreakpointsForDimension1=[-9.9,-9.7,-9.5,-9,-8.5,-8,-7.5,-7,7,7.5,8,8.5,9,9.5,9.7,9.9]  Table=[0,0.06,0.17,0.44,0.7,0.92,0.98,1,1,0.98,0.92,0.7,0.44,0.17,0.06,0]  ExtrapMethod=Clip  UseLastTableValue=on  InternalRulePriority=Speed  RndMeth=Simplest  InputSameDT=on
  Add : Sum
  Add1 : Sum
  Bus Selector2 : BusSelector  OutputSignals=y.ay
  Constant11 : Constant
  Constant12 : Constant  Value=0
  Constant2 : Constant  Value=0
  Constant3 : Constant
  Enabled Subsystem : Subsystem  TreatAsAtomicUnit=on
  Enabled Subsystem1 : Subsystem  TreatAsAtomicUnit=on
  Gain1 : Gain  Gain=-1
  Product{,1..3} (4 alike) : Product
  Saturation : Saturate  UpperLimit=par_VEH.Iz  LowerLimit=-par_VEH.Iz
  Saturation Dynamic : simulink/Discontinuities/Saturation Dynamic  OutMin=[]  OutMax=[]  OutDataTypeStr=Inherit: Same as second input  OutDataType=fixdt(1, 16)  OutScaling=2^-10  DoSatur=off
  Switch1 : Switch  Criteria=u2 > Threshold  Threshold=1
  Switch2 : Switch  Criteria=u2 > Threshold  Threshold=7.5
  Switch3 : Switch  Criteria=u2 > Threshold  Threshold=1
  M_z_desired : Outport
  wires:
  Switch3/1 -> Enabled Subsystem/Enable
  Constant12/1 -> Switch3/1
  Enabled Subsystem1/1(Out1) -> Switch3/2, Switch3/3
  Constant11/1 -> Enabled Subsystem1/1(In1)
  Switch2/1 -> Enabled Subsystem1/Enable
  Constant3/1 -> Switch2/1
  Constant2/1 -> Switch2/3
  Enabled Subsystem/1(Out1) -> Saturation Dynamic/1, Gain1/1
  Bus Selector2/1 -> Switch2/2, Product3/2, 1-D Lookup Table2/1, 1-D Lookup Table1/1, 1-D Lookup Table/1  "<ay>"
  Input/1 -> Bus Selector2/1
  M_z_FF/1 -> Enabled Subsystem/1(In1), Product/2, Saturation Dynamic/2
  1-D Lookup Table/1 -> Product/1
  Product/1 -> Add1/1
  Saturation Dynamic/1 -> Product2/2
  1-D Lookup Table2/1 -> Product1/2
  Product3/1 -> Switch1/2
  M_z_FB/1 -> Product1/1, Switch1/3, Product3/1
  Saturation/1 -> M_z_desired/1
  Product1/1 -> Switch1/1
  Product2/1 -> Add1/2
  Switch1/1 -> Add/1
  Add1/1 -> Add/2
  Gain1/1 -> Saturation Dynamic/3
  Add/1 -> Saturation/1
  1-D Lookup Table1/1 -> Product2/1

== system simulation/Vehicle/Antriebsstrang und Radmomentenverteilung/Batterie/Electrical battery cell model/Dynamic parameter set ==
  x_k : Inport  PortDimensions=[3 1]
  Ah to As : Gain  Gain=3600
  Bus Creator : BusCreator  Inputs=6
  C1 : Lookup_n-D  NumberOfTableDimensions=1  BreakpointsForDimension1=par_MDT.AUS.batt.Daten_Batteriemodell.BatPara.ECMPara.Dyn.EIS.SOCs  BreakpointsForDimension2=Bat_param.Dyn.C_rate  BreakpointsForDimension3=temperature_LTrange  Table=par_MDT.AUS.batt.Daten_Batteriemodell.BatPara.ECMPara.Dyn.EIS.C1  ExtrapMethod=Clip  UseLastTableValue=on  InternalRulePriority=Speed  RndMeth=Simplest  InputSameDT=on
  C2 : Lookup_n-D  NumberOfTableDimensions=1  BreakpointsForDimension1=par_MDT.AUS.batt.Daten_Batteriemodell.BatPara.ECMPara.Dyn.EIS.SOCs  BreakpointsForDimension2=Bat_param.Dyn.C_rate  BreakpointsForDimension3=temperature_LTrange  Table=par_MDT.AUS.batt.Daten_Batteriemodell.BatPara.ECMPara.Dyn.EIS.C2  ExtrapMethod=Clip  UseLastTableValue=on  InternalRulePriority=Speed  RndMeth=Simplest  InputSameDT=on
  Cell capacity : Constant  Value=par_MDT.AUS.batt.Daten_Batteriemodell.BatPara.ECMPara.CA
  R1 : Lookup_n-D  NumberOfTableDimensions=1  BreakpointsForDimension1=par_MDT.AUS.batt.Daten_Batteriemodell.BatPara.ECMPara.Dyn.EIS.SOCs  BreakpointsForDimension2=Bat_param.Dyn.C_rate  BreakpointsForDimension3=temperature_LTrange  Table=par_MDT.AUS.batt.Daten_Batteriemodell.BatPara.ECMPara.Dyn.EIS.R1  ExtrapMethod=Clip  UseLastTableValue=on  InternalRulePriority=Speed  RndMeth=Simplest  InputSameDT=on
  R2 : Lookup_n-D  NumberOfTableDimensions=1  BreakpointsForDimension1=par_MDT.AUS.batt.Daten_Batteriemodell.BatPara.ECMPara.Dyn.EIS.SOCs  BreakpointsForDimension2=Bat_param.Dyn.C_rate  BreakpointsForDimension3=temperature_LTrange  Table=par_MDT.AUS.batt.Daten_Batteriemodell.BatPara.ECMPara.Dyn.EIS.R2  ExtrapMethod=Clip  UseLastTableValue=on  InternalRulePriority=Speed  RndMeth=Simplest  InputSameDT=on
  R_0 : Lookup_n-D  NumberOfTableDimensions=1  BreakpointsForDimension1=par_MDT.AUS.batt.Daten_Batteriemodell.BatPara.ECMPara.Dyn.EIS.SOCs  BreakpointsForDimension2=Bat_param.Dyn.C_rate  BreakpointsForDimension3=temperature_LTrange  Table=par_MDT.AUS.batt.Daten_Batteriemodell.BatPara.ECMPara.Dyn.EIS.Rohm  ExtrapMethod=Clip  UseLastTableValue=on  InternalRulePriority=Speed  RndMeth=Simplest  InputSameDT=on
  Selector : Selector  InputPortWidth=3  IndexOptions=Index vector (dialog)  Indices=1  OutputSizes=1
  bat_param : Outport
  wires:
  Bus Creator/1 -> bat_param/1
  R1/1 -> Bus Creator/3  "R_1"
  Ah to As/1 -> Bus Creator/6  "C_N"
  C1/1 -> Bus Creator/1  "C_1"
  R2/1 -> Bus Creator/4  "R_2"
  C2/1 -> Bus Creator/2  "C_2"
  x_k/1 -> Selector/1
  Selector/1 -> R_0/1, R2/1, R1/1, C2/1, C1/1  "SOC"
  Cell capacity/1 -> Ah to As/1  "C_N"
  R_0/1 -> Bus Creator/5  "R_0"

== system simulation/Vehicle/Betriebsstrategie/Momentenverteilung_und_Schaltstrategie1/ASR/opt Schlupf ==
  mu_RF : Inport
  mu_LF : Inport  Port=2
  mu_RR : Inport  Port=3
  mu_LR : Inport  Port=4
  Fz_RF : Inport  Port=5
  Fz_LF : Inport  Port=6
  Fz_RR : Inport  Port=7
  Fz_LR : Inport  Port=8
  2-D Lookup Table{,1..3} (4 alike) : Lookup_n-D  BreakpointsForDimension1=par_ASR.mu  BreakpointsForDimension2=par_ASR.Fz  Table=par_ASR.Schlupf'  InternalRulePriority=Speed  RndMeth=Simplest  InputSameDT=on
  kappa_soll_RF : Outport
  kappa_soll_LF : Outport  Port=2
  kappa_soll_RR : Outport  Port=3
  kappa_soll_LR : Outport  Port=4
  wires:
  2-D Lookup Table/1 -> kappa_soll_RF/1
  mu_RF/1 -> 2-D Lookup Table/1
  Fz_RF/1 -> 2-D Lookup Table/2
  2-D Lookup Table1/1 -> kappa_soll_LF/1
  mu_LF/1 -> 2-D Lookup Table1/1
  Fz_LF/1 -> 2-D Lookup Table1/2
  2-D Lookup Table2/1 -> kappa_soll_RR/1
  mu_RR/1 -> 2-D Lookup Table2/1
  Fz_RR/1 -> 2-D Lookup Table2/2
  2-D Lookup Table3/1 -> kappa_soll_LR/1
  mu_LR/1 -> 2-D Lookup Table3/1
  Fz_LR/1 -> 2-D Lookup Table3/2

== system simulation/Vehicle/Betriebsstrategie/Momentenverteilung_und_Schaltstrategie1/Limitierungen gesamt (mit MVS Limits)/Aktuatoren und Delta TV ==
  Aktuator : Constant  Value=par_MDT.AUS.akt.OD_VA
  Aktuator1 : Constant  Value=0
  Aktuator10 : Constant  Value=par_MDT.AUS.akt.TS_VA
  Aktuator11 : Constant  Value=par_MDT.AUS.akt.TS_HA
  Aktuator3 : Constant  Value=par_MDT.AUS.akt.eTV_VA
  Aktuator4 : Constant  Value=par_MDT.AUS.akt.az_VA
  Aktuator5 : Constant  Value=par_MDT.AUS.akt.OD_HA
  Aktuator6 : Constant  Value=0
  Aktuator8 : Constant  Value=par_MDT.AUS.akt.eTV_HA
  Aktuator9 : Constant  Value=par_MDT.AUS.akt.az_HA
  Limit elektrisches Überlagerungsgetriebe : Constant  Value=595
  Limit mechanisches Überlagerungsgetriebe1 : Constant  Value=595
  Limit mechanisches Überlagerungsgetriebe2 : Constant  Value=595
  Limit mechanisches Überlagerungsgetriebe3 : Constant  Value=595
  Logical Operator : Logic  Operator=NOT  AllPortsSameDT=off  OutDataTypeStr=boolean
  Logical Operator1 : Logic  Operator=NOT  AllPortsSameDT=off  OutDataTypeStr=boolean
  TV Moment pro Achse : MATLAB Function  TreatAsAtomicUnit=on
  Zuweisung Aktuatoren : MATLAB Function  TreatAsAtomicUnit=on
  Delta_T_f : Outport
  Delta_T_r : Outport  Port=2
  A_f : Outport  Port=3
  A_r : Outport  Port=4
  wires:
  Zuweisung Aktuatoren/1(a_f) -> A_f/1, TV Moment pro Achse/6(a_f)
  Aktuator9/1 -> Logical Operator1/1
  Aktuator8/1 -> Zuweisung Aktuatoren/9(A9)
  Aktuator11/1 -> Zuweisung Aktuatoren/8(A8)
  Aktuator6/1 -> Zuweisung Aktuatoren/7(A7)
  Aktuator5/1 -> Zuweisung Aktuatoren/6(A6)
  Aktuator4/1 -> Logical Operator/1
  Aktuator3/1 -> Zuweisung Aktuatoren/4(A4)
  Aktuator10/1 -> Zuweisung Aktuatoren/3(A3)
  Aktuator1/1 -> Zuweisung Aktuatoren/2(A2)
  Aktuator/1 -> Zuweisung Aktuatoren/1(A1)
  Zuweisung Aktuatoren/2(a_r) -> A_r/1, TV Moment pro Achse/7(a_r)
  TV Moment pro Achse/1(Delta_T_f) -> Delta_T_f/1
  TV Moment pro Achse/2(Delta_T_r) -> Delta_T_r/1
  Limit elektrisches Überlagerungsgetriebe/1 -> TV Moment pro Achse/1(L1)
  Limit mechanisches Überlagerungsgetriebe1/1 -> TV Moment pro Achse/2(L2)
  Limit mechanisches Überlagerungsgetriebe2/1 -> TV Moment pro Achse/3(L3)
  Limit mechanisches Überlagerungsgetriebe3/1 -> TV Moment pro Achse/4(L4)
  Logical Operator/1 -> Zuweisung Aktuatoren/5(A5)
  Logical Operator1/1 -> Zuweisung Aktuatoren/10(A10)

== system simulation/Vehicle/Betriebsstrategie/Momentenverteilung_und_Schaltstrategie1/Motor Limits/Limit_F_lb ==
  Raddrehzahl : Inport
  Drehmoment : Product
  Drehzahl : Product
  Getriebeuebersetzung : Constant  Value=par_MDT.VA.trans.i_gears
  Getriebewirkungsgrad : Constant  Value=par_MDT.VA.trans.wkg
  M_Reku : Lookup_n-D  NumberOfTableDimensions=1  BreakpointsForDimension1=par_MDT.VA.em.MaxGeneratorTrqCurve_w  Table=par_MDT.VA.em.MaxGeneratorTrqCurve_M  ExtrapMethod=Clip  UseLastTableValue=on  InternalRulePriority=Speed  RndMeth=Simplest  InputSameDT=on
  MinMax : MinMax  Function=max
  Rueckrechnung : Product
  Moment : Outport
  wires:
  Drehzahl/1 -> M_Reku/1
  Getriebeuebersetzung/1 -> Drehzahl/2, Drehmoment/2
  Raddrehzahl/1 -> Drehzahl/1
  M_Reku/1 -> Drehmoment/1
  Drehmoment/1 -> Rueckrechnung/1
  Rueckrechnung/1 -> MinMax/1
  Getriebewirkungsgrad/1 -> Rueckrechnung/2
  MinMax/1 -> Moment/1

== system simulation/Vehicle/Betriebsstrategie/Momentenverteilung_und_Schaltstrategie1/Motor Limits/Limit_F_ub ==
  Raddrehzahl : Inport
  Drehmoment : Product
  Drehzahl : Product
  Getriebeuebersetzung : Constant  Value=par_MDT.VA.trans.i_gears
  Getriebewirkungsgrad : Constant  Value=par_MDT.VA.trans.wkg
  M_Antr : Lookup_n-D  NumberOfTableDimensions=1  BreakpointsForDimension1=par_MDT.VA.em.MaxMotorTrqCurve_w  Table=par_MDT.VA.em.MaxMotorTrqCurve_M  ExtrapMethod=Clip  UseLastTableValue=on  InternalRulePriority=Speed  RndMeth=Simplest  InputSameDT=on
  MinMax : MinMax  Function=max
  Rueckrechnung : Product
  Moment : Outport
  wires:
  Drehzahl/1 -> M_Antr/1
  Getriebeuebersetzung/1 -> Drehzahl/2, Drehmoment/2
  Raddrehzahl/1 -> Drehzahl/1
  M_Antr/1 -> Drehmoment/1
  Drehmoment/1 -> Rueckrechnung/1
  Rueckrechnung/1 -> MinMax/1
  Getriebewirkungsgrad/1 -> Rueckrechnung/2
  MinMax/1 -> Moment/1

== system simulation/Vehicle/Betriebsstrategie/Momentenverteilung_und_Schaltstrategie1/Motor Limits/Limit_LF_lb ==
  Raddrehzahl : Inport
  Drehmoment : Product
  Drehzahl : Product
  Getriebeuebersetzung : Constant  Value=par_MDT.VA.trans.i_gears
  Getriebewirkungsgrad : Constant  Value=par_MDT.VA.trans.wkg
  M_Reku : Lookup_n-D  NumberOfTableDimensions=1  BreakpointsForDimension1=par_MDT.VA.em.MaxGeneratorTrqCurve_w  Table=par_MDT.VA.em.MaxGeneratorTrqCurve_M  ExtrapMethod=Clip  UseLastTableValue=on  InternalRulePriority=Speed  RndMeth=Simplest  InputSameDT=on
  MinMax : MinMax  Function=max
  Rueckrechnung : Product
  Moment : Outport
  wires:
  Drehzahl/1 -> M_Reku/1
  Getriebeuebersetzung/1 -> Drehzahl/2, Drehmoment/2
  Raddrehzahl/1 -> Drehzahl/1
  M_Reku/1 -> Drehmoment/1
  Drehmoment/1 -> Rueckrechnung/1
  Rueckrechnung/1 -> MinMax/1
  Getriebewirkungsgrad/1 -> Rueckrechnung/2
  MinMax/1 -> Moment/1

== system simulation/Vehicle/Betriebsstrategie/Momentenverteilung_und_Schaltstrategie1/Motor Limits/Limit_LF_ub ==
  Raddrehzahl : Inport
  Drehmoment : Product
  Drehzahl : Product
  Getriebeuebersetzung : Constant  Value=par_MDT.VA.trans.i_gears
  Getriebewirkungsgrad : Constant  Value=par_MDT.VA.trans.wkg
  M_Antr : Lookup_n-D  NumberOfTableDimensions=1  BreakpointsForDimension1=par_MDT.VA.em.MaxMotorTrqCurve_w  Table=par_MDT.VA.em.MaxMotorTrqCurve_M  ExtrapMethod=Clip  UseLastTableValue=on  InternalRulePriority=Speed  RndMeth=Simplest  InputSameDT=on
  MinMax : MinMax  Function=max
  Rueckrechnung : Product
  Moment : Outport
  wires:
  Drehzahl/1 -> M_Antr/1
  Getriebeuebersetzung/1 -> Drehzahl/2, Drehmoment/2
  Raddrehzahl/1 -> Drehzahl/1
  M_Antr/1 -> Drehmoment/1
  Drehmoment/1 -> Rueckrechnung/1
  Rueckrechnung/1 -> MinMax/1
  Getriebewirkungsgrad/1 -> Rueckrechnung/2
  MinMax/1 -> Moment/1

== system simulation/Vehicle/Betriebsstrategie/Momentenverteilung_und_Schaltstrategie1/Motor Limits/Limit_LR_lb ==
  Raddrehzahl : Inport
  Drehmoment : Product
  Drehzahl : Product
  Getriebeuebersetzung : Constant  Value=par_MDT.HA.trans.i_gears
  Getriebewirkungsgrad : Constant  Value=par_MDT.HA.trans.wkg
  M_Reku : Lookup_n-D  NumberOfTableDimensions=1  BreakpointsForDimension1=par_MDT.HA.em.MaxGeneratorTrqCurve_w  Table=par_MDT.HA.em.MaxGeneratorTrqCurve_M  ExtrapMethod=Clip  UseLastTableValue=on  InternalRulePriority=Speed  RndMeth=Simplest  InputSameDT=on
  MinMax : MinMax  Function=max
  Rueckrechnung : Product
  Moment : Outport
  wires:
  Drehzahl/1 -> M_Reku/1
  Getriebeuebersetzung/1 -> Drehzahl/2, Drehmoment/2
  Raddrehzahl/1 -> Drehzahl/1
  M_Reku/1 -> Drehmoment/1
  Drehmoment/1 -> Rueckrechnung/1
  Rueckrechnung/1 -> MinMax/1
  Getriebewirkungsgrad/1 -> Rueckrechnung/2
  MinMax/1 -> Moment/1

== system simulation/Vehicle/Betriebsstrategie/Momentenverteilung_und_Schaltstrategie1/Motor Limits/Limit_LR_ub ==
  Raddrehzahl : Inport
  Drehmoment : Product
  Drehzahl : Product
  Getriebeuebersetzung : Constant  Value=par_MDT.HA.trans.i_gears
  Getriebewirkungsgrad : Constant  Value=par_MDT.HA.trans.wkg
  M_Antr : Lookup_n-D  NumberOfTableDimensions=1  BreakpointsForDimension1=par_MDT.HA.em.MaxMotorTrqCurve_w  Table=par_MDT.HA.em.MaxMotorTrqCurve_M  ExtrapMethod=Clip  UseLastTableValue=on  InternalRulePriority=Speed  RndMeth=Simplest  InputSameDT=on
  MinMax : MinMax  Function=max
  Rueckrechnung : Product
  Moment : Outport
  wires:
  Drehzahl/1 -> M_Antr/1
  Getriebeuebersetzung/1 -> Drehzahl/2, Drehmoment/2
  Raddrehzahl/1 -> Drehzahl/1
  M_Antr/1 -> Drehmoment/1
  Drehmoment/1 -> Rueckrechnung/1
  Rueckrechnung/1 -> MinMax/1
  Getriebewirkungsgrad/1 -> Rueckrechnung/2
  MinMax/1 -> Moment/1

== system simulation/Vehicle/Betriebsstrategie/Momentenverteilung_und_Schaltstrategie1/Motor Limits/Limit_RF_lb ==
  Raddrehzahl : Inport
  Drehmoment : Product
  Drehzahl : Product
  Getriebeuebersetzung : Constant  Value=par_MDT.VA.trans.i_gears
  Getriebewirkungsgrad : Constant  Value=par_MDT.VA.trans.wkg
  M_Reku : Lookup_n-D  NumberOfTableDimensions=1  BreakpointsForDimension1=par_MDT.VA.em.MaxGeneratorTrqCurve_w  Table=par_MDT.VA.em.MaxGeneratorTrqCurve_M  ExtrapMethod=Clip  UseLastTableValue=on  InternalRulePriority=Speed  RndMeth=Simplest  InputSameDT=on
  MinMax : MinMax  Function=max
  Rueckrechnung : Product
  Moment : Outport
  wires:
  Drehzahl/1 -> M_Reku/1
  Getriebeuebersetzung/1 -> Drehzahl/2, Drehmoment/2
  Raddrehzahl/1 -> Drehzahl/1
  M_Reku/1 -> Drehmoment/1
  Drehmoment/1 -> Rueckrechnung/1
  Rueckrechnung/1 -> MinMax/1
  Getriebewirkungsgrad/1 -> Rueckrechnung/2
  MinMax/1 -> Moment/1

== system simulation/Vehicle/Betriebsstrategie/Momentenverteilung_und_Schaltstrategie1/Motor Limits/Limit_RF_ub ==
  Raddrehzahl : Inport
  Drehmoment : Product
  Drehzahl : Product
  Getriebeuebersetzung : Constant  Value=par_MDT.VA.trans.i_gears
  Getriebewirkungsgrad : Constant  Value=par_MDT.VA.trans.wkg
  M_Antr : Lookup_n-D  NumberOfTableDimensions=1  BreakpointsForDimension1=par_MDT.VA.em.MaxMotorTrqCurve_w  Table=par_MDT.VA.em.MaxMotorTrqCurve_M  ExtrapMethod=Clip  UseLastTableValue=on  InternalRulePriority=Speed  RndMeth=Simplest  InputSameDT=on
  MinMax : MinMax  Function=max
  Rueckrechnung : Product
  Moment : Outport
  wires:
  Drehzahl/1 -> M_Antr/1
  Getriebeuebersetzung/1 -> Drehzahl/2, Drehmoment/2
  Raddrehzahl/1 -> Drehzahl/1
  M_Antr/1 -> Drehmoment/1
  Drehmoment/1 -> Rueckrechnung/1
  Rueckrechnung/1 -> MinMax/1
  Getriebewirkungsgrad/1 -> Rueckrechnung/2
  MinMax/1 -> Moment/1

== system simulation/Vehicle/Betriebsstrategie/Momentenverteilung_und_Schaltstrategie1/Motor Limits/Limit_RR_lb ==
  Raddrehzahl : Inport
  Drehmoment : Product
  Drehzahl : Product
  Getriebeuebersetzung : Constant  Value=par_MDT.HA.trans.i_gears
  Getriebewirkungsgrad : Constant  Value=par_MDT.HA.trans.wkg
  M_Reku : Lookup_n-D  NumberOfTableDimensions=1  BreakpointsForDimension1=par_MDT.HA.em.MaxGeneratorTrqCurve_w  Table=par_MDT.HA.em.MaxGeneratorTrqCurve_M  ExtrapMethod=Clip  UseLastTableValue=on  InternalRulePriority=Speed  RndMeth=Simplest  InputSameDT=on
  MinMax : MinMax  Function=max
  Rueckrechnung : Product
  Moment : Outport
  wires:
  Drehzahl/1 -> M_Reku/1
  Getriebeuebersetzung/1 -> Drehzahl/2, Drehmoment/2
  Raddrehzahl/1 -> Drehzahl/1
  M_Reku/1 -> Drehmoment/1
  Drehmoment/1 -> Rueckrechnung/1
  Rueckrechnung/1 -> MinMax/1
  Getriebewirkungsgrad/1 -> Rueckrechnung/2
  MinMax/1 -> Moment/1
